simulink model "ZSB"  (Simulink 8.3)
settings: Solver=ode4  StartTime=0.0  StopTime=4  FixedStep=0.00001  RelTol=1e-3
undefined symbols (not defined in the file): sigbuilder_block
settings Model: Creator=Chan Hwaiwing  LastModifiedBy=shubo
settings DataIOCC: SignalLoggingSaveFormat=Dataset
settings DebuggingCC: UnderspecifiedInitializationDetection=Simplified  MergeDetectMultiDrivingBlocksExec=error  FrameProcessingCompatibilityMsg=error  StateNameClashWarn=none
settings GRTTargetCC: CombineOutputUpdateFcns=on  GRTInterface=off
settings ConfigComp: CovCompData="CovMetricSettings\t  dw"  CovFilter=CovHTMLOptions  CovHtmlReporting=on  CovSaveCumulativeToWorkspaceVar=on  CovSaveSingleToWorkspaceVar=on  CovModelRefExcluded="CovExternalEMLEnable\t  off"  CovSFcnEnable=off

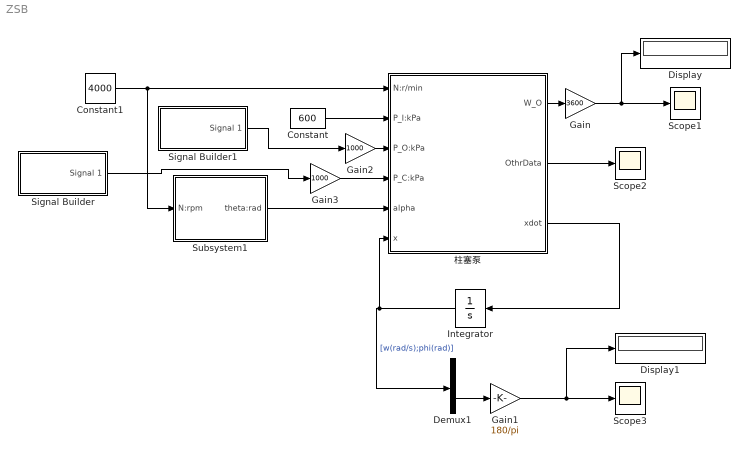
== system ZSB ==
  Constant : Constant  Value=600
  Constant1 : Constant  Value=4000
  Demux1 : Demux  Outputs=2
  Display : Display
  Display1 : Display
  Gain : Gain  Gain=3600
  Gain1 : Gain  Gain=180/pi
  Gain2 : Gain  Gain=1000
  Gain3 : Gain  Gain=1000
  Integrator : Integrator  InitialCondition=[0 14/180*pi]  LimitOutput=on  UpperSaturationLimit=[inf 14/180*pi]  LowerSaturationLimit=[-inf 0/180*pi ]
  Scope1 : Scope
      settings: YMin=3565  YMax=3635
  Scope2 : Scope
  Scope3 : Scope
      settings: TimeRange=1  YMin=12.78  YMax=12.7885  SaveName=ScopeData2
  Signal Builder : Subsystem  Tag=STV Subsys  LoadFcn=sigbuilder_block('load');  StartFcn=sigbuilder_block('start');  StopFcn=sigbuilder_block('stop');  ClipboardFcn=sigbuilder_block('clipboard');  mask(Sigbuilder block){}
      mask help: Simulink:masks:SigbuilderBlock_MD
      mask init:
      | if ~strcmp(get_param(bdroot(gcbh),'SimulationStatus'),'stopped') tuvar = sigbuilder_block('maskInit'); end
      settings: CopyFcn=sigbuilder_block('copy');  DeleteFcn=sigbuilder_block('delete');  ModelCloseFcn=sigbuilder_block('modelClose');  PreSaveFcn=sigbuilder_block('preSave');  PauseFcn=sigbuilder_block('pause');  ContinueFcn=sigbuilder_block('continue');  NameChangeFcn=sigbuilder_block('namechange');  OpenFcn=sigbuilder_block('open',[-1280.25 6 1280.25 469.5 ]);  CloseFcn=sigbuilder_block('close');
      mask Display: plot(0, 0, 100, 100,[2, 2, 32, 32, 2], [68, 8, 8, 68, 68],[32, 2], [38, 38], [32, 19, 2],[53, 60, 44], [32, 17, 17, 2],[16, 16, 31, 31]);txt = getActiveGroup(gcbh);text(2, 100, txt,'verticalAlignment', 'top');
  Signal Builder1 : Subsystem  Tag=STV Subsys  LoadFcn=sigbuilder_block('load');  StartFcn=sigbuilder_block('start');  StopFcn=sigbuilder_block('stop');  ClipboardFcn=sigbuilder_block('clipboard');  mask(Sigbuilder block){}
      mask help: Simulink:masks:SigbuilderBlock_MD
      mask init:
      | if ~strcmp(get_param(bdroot(gcbh),'SimulationStatus'),'stopped') tuvar = sigbuilder_block('maskInit'); end
      settings: CopyFcn=sigbuilder_block('copy');  DeleteFcn=sigbuilder_block('delete');  ModelCloseFcn=sigbuilder_block('modelClose');  PreSaveFcn=sigbuilder_block('preSave');  PauseFcn=sigbuilder_block('pause');  ContinueFcn=sigbuilder_block('continue');  NameChangeFcn=sigbuilder_block('namechange');  OpenFcn=sigbuilder_block('open',[-1280.25 129 1280.25 631.5 ]);  CloseFcn=sigbuilder_block('close');
      mask Display: plot(0, 0, 100, 100,[2, 2, 32, 32, 2], [68, 8, 8, 68, 68],[32, 2], [38, 38], [32, 19, 2],[53, 60, 44], [32, 17, 17, 2],[16, 16, 31, 31]);txt = getActiveGroup(gcbh);text(2, 100, txt,'verticalAlignment', 'top');
  Subsystem1 : Subsystem
  柱塞泵 : Subsystem  AncestorBlock=HMMtoolbox/泵类/ZSB  mask(柱塞泵){RHO=850, mode=脉动模式, L_ZSBHX=35, D_ZSBZS=52, A_ZSBZS=14.5*14.5*pi/4, ETA_V=1, M_ZS=0.05, Z_ZSBZS=9, BETA_ZSBZS=0/180*pi, A_ZSBTJ=[pi*(18.7^2)/4, pi*(18.7^2)/4], L_ZSBTJ=[57.146 68.907 35.796 304.493 159.595]*0.7, k=50000, BETA_ZSBSD=0/180*pi, L_x0=24, J_ZSBXP=0.34*0.2, KD=7.65*1}
      mask prompts: RHO "RHO(标准状态下，油液密度kg/m^3)"; mode "计算模式"; L_ZSBHX "L_HX(等效滑靴厚度mm)"; D_ZSBZS "D_ZS(柱塞轴线在缸体的分布圆直径mm)"; A_ZSBZS "A_ZS(柱塞截面面积mm^2)"; ETA_V "ETA_V(容积效率)"; M_ZS "M_ZS(柱塞质量kg)"; Z_ZSBZS "Z_ZS(柱塞数量)"; BETA_ZSBZS "BETA_ZS(柱塞安装角rad)"; A_ZSBTJ "A_TJ(面积参数向量mm^2)"; L_ZSBTJ "L_TJ(距离参数向量mm)"; k "k(弹簧弹性模量N/m)"; BETA_ZSBSD "BETA_SD(随动活塞安装角rad)"; L_x0 "L_x0(随动活塞初始位置mm)"; J_ZSBXP "J_XP(斜盘绕斜盘轴的转动惯量kg·m^2)"; KD "KD(斜盘转动阻力系数N·m·s/rad)"
      mask TypeOptions mode: 脉动模式 | 平均模式
      mask DialogControl DescTextVar Prompt: 填入相关参数
  wires:
  Subsystem1/1(theta:rad) -> 柱塞泵/5(alpha)
  柱塞泵/3(xdot) -> Integrator/1
  柱塞泵/2(OthrData) -> Scope2/1
  Constant/1 -> 柱塞泵/2(P_I:kPa)
  Constant1/1 -> Subsystem1/1(N:rpm), 柱塞泵/1(N:r/min)
  柱塞泵/1(W_O) -> Gain/1
  Demux1/2 -> Gain1/1
  Gain/1 -> Display/1, Scope1/1
  Gain1/1 -> Display1/1, Scope3/1
  Integrator/1 -> 柱塞泵/6(x), Demux1/1  "[w(rad/s);phi(rad)]"
  Signal Builder/1(Signal 1) -> Gain3/1
  Signal Builder1/1(Signal 1) -> Gain2/1
  Gain2/1 -> 柱塞泵/3(P_O:kPa)
  Gain3/1 -> 柱塞泵/4(P_C:kPa)

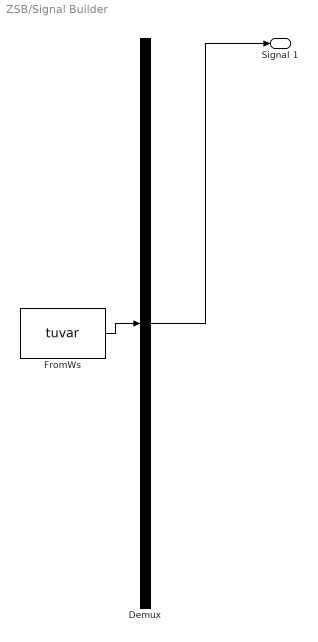
== system ZSB/Signal Builder ==
  Demux : Demux  Tag=STV Demux  Outputs=1
  FromWs : FromWorkspace  Tag=STV FromWs  VariableName=tuvar  SampleTime=0  SigBuilderData=DataTag0  VnvData=DataTag1
      SigBuilderData=|
      | common.afterFinalStr = 'Extrapolate'
      | common.sampleTime = 0
      | dataSet.timeRange = [0 4]
      | dataSet.name = 'Group 1'
      | sbobj.Groups.Name = 'Group 1'
      | sbobj.Groups.Signals.Name = 'Signal 1'
      | sbobj.Groups.Signals.XData = [0 1 1 2 2 3 3 4]
      | sbobj.Groups.Signals.YData = [1 1 2.5 2.5 4 4 5.4 5.4]
      | sbobj.Groups.TimeRange = [0 4]
  Signal 1 : Outport  Tag=STV Outport
  wires:
  Demux/1 -> Signal 1/1
  FromWs/1 -> Demux/1

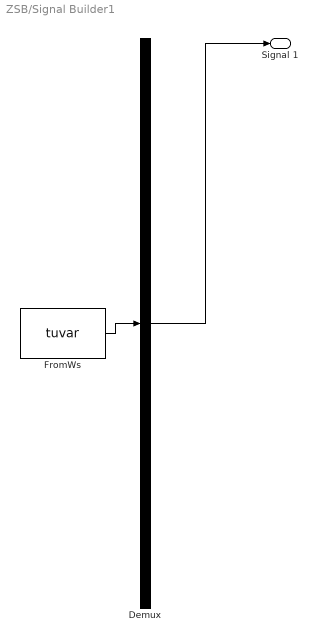
== system ZSB/Signal Builder1 ==
  Demux : Demux  Tag=STV Demux  Outputs=1
  FromWs : FromWorkspace  Tag=STV FromWs  VariableName=tuvar  SampleTime=0  SigBuilderData=DataTag2  VnvData=DataTag3
      SigBuilderData=|
      | common.afterFinalStr = 'Extrapolate'
      | common.sampleTime = 0
      | dataSet.timeRange = [0 4]
      | dataSet.name = 'Group 1'
      | sbobj.Groups.Name = 'Group 1'
      | sbobj.Groups.Signals.Name = 'Signal 1'
      | sbobj.Groups.Signals.XData = [0 1 1 2 2 3 3 4]
      | sbobj.Groups.Signals.YData = [8.65 8.65 12.7 12.7 16.8 16.8 20.6 20.6]
      | sbobj.Groups.TimeRange = [0 4]
  Signal 1 : Outport  Tag=STV Outport
  wires:
  Demux/1 -> Signal 1/1
  FromWs/1 -> Demux/1

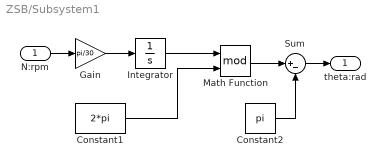
== system ZSB/Subsystem1 ==
  N:rpm : Inport
  Constant1 : Constant  Value=2*pi
  Constant2 : Constant  Value=pi
  Gain : Gain  Gain=pi/30
  Integrator : Integrator
  Math Function : Math  Operator=mod  SaturateOnIntegerOverflow=on
  Sum : Sum  Inputs=|+-
  theta:rad : Outport
  wires:
  Math Function/1 -> Sum/1
  N:rpm/1 -> Gain/1
  Constant1/1 -> Math Function/2
  Integrator/1 -> Math Function/1
  Gain/1 -> Integrator/1
  Sum/1 -> theta:rad/1
  Constant2/1 -> Sum/2

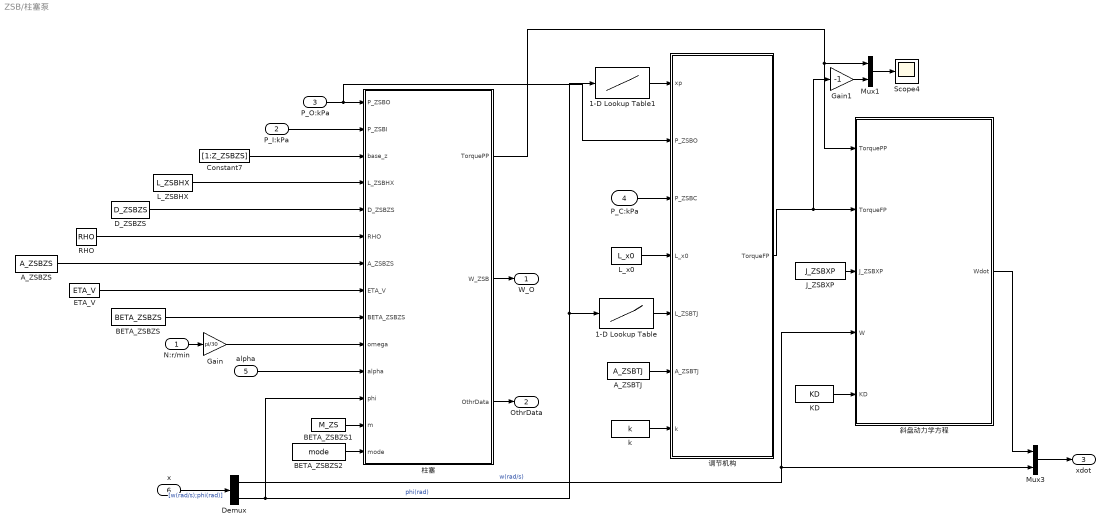
== system ZSB/柱塞泵 ==
  N:r/min : Inport
  P_I:kPa : Inport  Port=2
  P_O:kPa : Inport  Port=3
  P_C:kPa : Inport  Port=4
  alpha : Inport  Port=5
  x : Inport  Port=6
  1-D Lookup Table : Lookup_n-D  NumberOfTableDimensions=1  BreakpointsForDimension1=[0 14/180*pi]  Table=[60 60]  InternalRulePriority=Speed  RndMeth=Simplest  InputSameDT=on
  1-D Lookup Table1 : Lookup_n-D  NumberOfTableDimensions=1  BreakpointsForDimension1=[0 14/180*pi]  Table=[0 13.8]  InternalRulePriority=Speed  RndMeth=Simplest  InputSameDT=on
  A_ZSBTJ : Constant  Value=A_ZSBTJ
  A_ZSBZS : Constant  Value=A_ZSBZS
  BETA_ZSBZS : Constant  Value=BETA_ZSBZS
  BETA_ZSBZS1 : Constant  Value=M_ZS
  BETA_ZSBZS2 : Constant  Value=mode
  Constant7 : Constant  Value=[1:Z_ZSBZS]
  D_ZSBZS : Constant  Value=D_ZSBZS
  Demux : Demux  Outputs=2
  ETA_V : Constant  Value=ETA_V
  Gain : Gain  Gain=pi/30
  Gain1 : Gain  Gain=-1
  J_ZSBXP : Constant  Value=J_ZSBXP
  KD : Constant  Value=KD
  L_ZSBHX : Constant  Value=L_ZSBHX
  L_x0 : Constant  Value=L_x0
  Mux1 : Mux  Inputs=2
  Mux3 : Mux  Inputs=2
  RHO : Constant  Value=RHO
  Scope4 : Scope
      settings: YMin=-100  SaveName=ScopeData4
  k : Constant  Value=k
  斜盘动力学方程 : MATLAB Function  TreatAsAtomicUnit=on
  柱塞 : MATLAB Function  TreatAsAtomicUnit=on
  调节机构 : MATLAB Function  TreatAsAtomicUnit=on
  W_O : Outport
  OthrData : Outport  Port=2
  xdot : Outport  Port=3
  wires:
  x/1 -> Demux/1  "[w(rad/s);phi(rad)]"
  斜盘动力学方程/1(Wdot) -> Mux3/1
  Mux3/1 -> xdot/1
  柱塞/3(OthrData) -> OthrData/1
  alpha/1 -> 柱塞/11(alpha)
  J_ZSBXP/1 -> 斜盘动力学方程/3(J_ZSBXP)
  A_ZSBTJ/1 -> 调节机构/6(A_ZSBTJ)
  BETA_ZSBZS/1 -> 柱塞/9(BETA_ZSBZS)
  ETA_V/1 -> 柱塞/8(ETA_V)
  D_ZSBZS/1 -> 柱塞/5(D_ZSBZS)
  Demux/1 -> 斜盘动力学方程/4(W), Mux3/2  "w(rad/s)"
  柱塞/2(W_ZSB) -> W_O/1
  k/1 -> 调节机构/7(k)
  柱塞/1(TorquePP) -> Mux1/1, 斜盘动力学方程/1(TorquePP)
  L_x0/1 -> 调节机构/4(L_x0)
  Gain/1 -> 柱塞/10(omega)
  P_O:kPa/1 -> 调节机构/2(P_ZSBO), 柱塞/1(P_ZSBO)
  L_ZSBHX/1 -> 柱塞/4(L_ZSBHX)
  RHO/1 -> 柱塞/6(RHO)
  Constant7/1 -> 柱塞/3(base_z)
  A_ZSBZS/1 -> 柱塞/7(A_ZSBZS)
  N:r/min/1 -> Gain/1
  P_C:kPa/1 -> 调节机构/3(P_ZSBC)
  P_I:kPa/1 -> 柱塞/2(P_ZSBI)
  KD/1 -> 斜盘动力学方程/5(KD)
  BETA_ZSBZS1/1 -> 柱塞/13(m)
  BETA_ZSBZS2/1 -> 柱塞/14(mode)
  Demux/2 -> 1-D Lookup Table1/1, 1-D Lookup Table/1, 柱塞/12(phi)  "phi(rad)"
  1-D Lookup Table/1 -> 调节机构/5(L_ZSBTJ)
  1-D Lookup Table1/1 -> 调节机构/1(xp)
  Mux1/1 -> Scope4/1
  调节机构/1(TorqueFP) -> 斜盘动力学方程/2(TorqueFP), Gain1/1
  Gain1/1 -> Mux1/2

== matlab function 柱塞泵/柱塞 ==
  data: P_ZSBO input double; P_ZSBI input double; base_z input double; L_ZSBHX input double; D_ZSBZS input double; RHO input double; A_ZSBZS input double; ETA_V input double; BETA_ZSBZS input double; omega input double; alpha input double; TorquePP output double; W_ZSB output double; OthrData output double; phi input double; m input double; mode input double
function [ TorquePP, W_ZSB, OthrData ] = Plunger_Pump(P_ZSBO,  P_ZSBI,  base_z, L_ZSBHX, D_ZSBZS, RHO, A_ZSBZS, ETA_V,BETA_ZSBZS,omega,alpha,phi, m, mode )
r=D_ZSBZS/2;
z = length( base_z );
S_max = 2 * r * tan( phi );

if ( mode == 1 )
    
    alpha_tab =  alpha + base_z * 2 * pi / z;
    v_tab = -r * sin( alpha_tab ) * tan( phi ) * omega;
    l_tab = r * cos( alpha_tab ) / cos( phi ) + L_ZSBHX * tan( phi );

    p_tab = base_z;
    for i = 1 : z
        if ( alpha_tab( i ) >= pi )
            alpha_tab( i ) =  alpha_tab( i ) - 2 * pi;
        end
        if ( alpha_tab( i ) < 0 )
            p_tab( i ) = P_ZSBO;
        else
            p_tab( i ) = P_ZSBI;
            v_tab( i ) = 0;
        end
    end
    f1_tab = A_ZSBZS * p_tab / cos( phi );
    f2_tab = - r * m * tan( phi ) * omega * omega * cos( alpha_tab );
    f_tab = f1_tab + f2_tab;
    m_tab = l_tab .* f_tab * 1e-6;

    TorquePP = -sum( m_tab ); 
    q_tab = A_ZSBZS * ETA_V*cos(BETA_ZSBZS) * v_tab * RHO * 1e-9; 
    W_ZSB = sum( q_tab );
    OthrData = [ S_max, v_tab( z ), q_tab( z ), l_tab( z ), f_tab( z ), m_tab( z ) ];

else

    TorqueLG = 0.5*r*r*z*m*tan(phi)*omega*omega/cos(phi);
    TorqueYY = -0.5*z*L_ZSBHX*tan(phi)*A_ZSBZS*(P_ZSBO+P_ZSBI)/cos(phi);
    TorquePP = (TorqueYY + TorqueLG) * 1e-6;
    W_ZSB = RHO * ETA_V *cos(BETA_ZSBZS)* A_ZSBZS * S_max * z * omega * 0.5 / pi * 1e-9;
    OthrData = [ S_max, 0, 0, 0, 0, 0 ];
end

end

== matlab function 柱塞泵/调节机构 ==
  data: xp input double; P_ZSBO input double; TorqueFP output double; P_ZSBC input double; L_x0 input double; L_ZSBTJ input double; A_ZSBTJ input double; k input double
function TorqueFP  = TJ( xp, P_ZSBO, P_ZSBC, L_x0, L_ZSBTJ, A_ZSBTJ, k )

%计算随动活塞杆上的作用力
Pleft = P_ZSBO * 1e3;%kPa
Pright = Pleft-P_ZSBC * 1e3;%kPa
Fleft = Pleft * A_ZSBTJ(1) * 1e-6;%N
Fright = Pright * A_ZSBTJ(2) * 1e-6;%N
Fs = k * (L_x0 - xp) * 1e-3;
Fsui = Fs - Fright + Fleft;

%计算随动活塞杆力对斜盘作用力矩
TorqueFP = Fsui*L_ZSBTJ*1e-3;

end

== matlab function 柱塞泵/斜盘动力学方程 ==
  data: TorquePP input double; Wdot output double; TorqueFP input double; J_ZSBXP input double; W input double; KD input double
function Wdot = DL(TorquePP,TorqueFP,J_ZSBXP,W, KD) 

    Torq_Net = TorquePP + TorqueFP - W * KD;
    Wdot =  Torq_Net / J_ZSBXP;
end
